simulink model "Day16"  (R2024b)
settings: Solver=VariableStepAuto  StartTime=0.0  StopTime=10.0  RelTol=1e-3
settings Model: Creator=jun_mac  LastModifiedBy=jun_mac

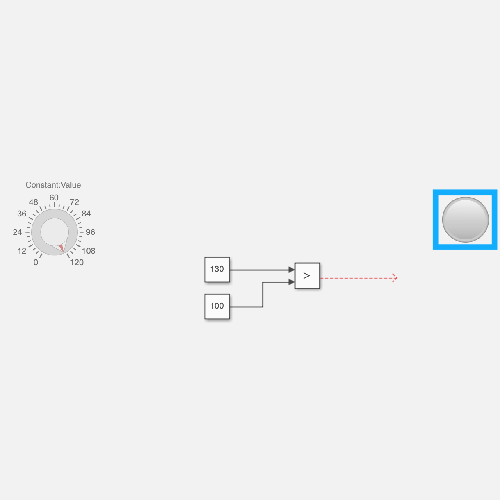
[thumbnail: Simulink's stored preview of the top-level diagram]
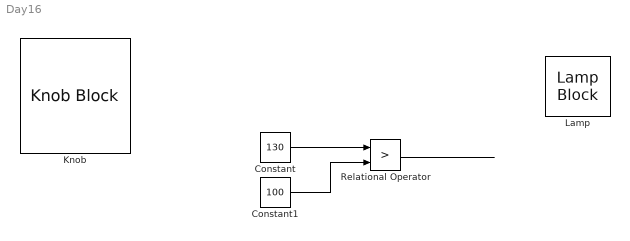
== system Day16 ==
  Constant : Constant  Value=130
  Constant1 : Constant  Value=100
  Knob : KnobBlock  ScaleMax=120
  Lamp : LampBlock  LabelPosition=Hide
  Relational Operator : RelationalOperator  Operator=>  OutDataTypeStr=boolean  RndMeth=Simplest  InputSameDT=off
  wires:
  Constant1/1 -> Relational Operator/2
  Constant/1 -> Relational Operator/1
  Relational Operator/1 -> ?
